simulink model "testFrame_ADCRawToIab"  (R2020b)
settings: Solver=VariableStepAuto  StartTime=0.0  StopTime=10.0  RelTol=1e-3
settings Model: Creator=unix  LastModifiedBy=unix

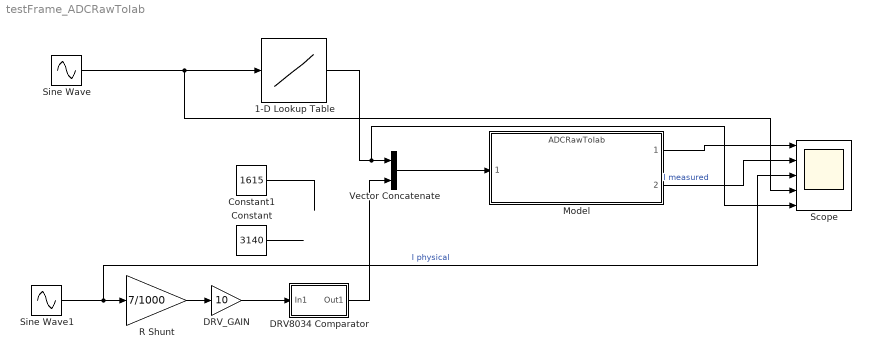
== system testFrame_ADCRawToIab ==
  1-D Lookup Table : Lookup_n-D  NumberOfTableDimensions=1  LookupTableObject=''  BreakpointsForDimension1=[0 3.3]  BreakpointsForDimension1FirstPoint=10  BreakpointsForDimension2FirstPoint=10  BreakpointsForDimension1Spacing=12  BreakpointsForDimension2Spacing=12  Table=[0 4096]  ExtrapMethod=Clip  DiagnosticForOutOfRangeInput=Error  InternalRulePriority=Speed  OutDataTypeStr=Inherit: Inherit via back propagation  RndMeth=Simplest  InputSameDT=on
  Constant : Constant  Value=3140  OutDataTypeStr=uint16
  Constant1 : Constant  Value=1615  OutDataTypeStr=uint16
  DRV8034 Comparator : Subsystem
  DRV_GAIN : Gain  Gain=10
  Model : ModelReference  ModelNameDialog=ADCRawToIab.slx  ModelReferenceVersion=3.1
  R Shunt : Gain  Gain=7/1000
  Scope : Scope  NumInputPorts=5
  Sine Wave : Sin  Amplitude=1.65  Bias=1.65  Frequency=50  SampleTime=0
  Sine Wave1 : Sin  Amplitude=22  Frequency=50  SampleTime=0
  Vector Concatenate : Concatenate
  wires:
  Sine Wave/1 -> Scope/4, 1-D Lookup Table/1
  Vector Concatenate/1 -> Model/1
  Model/1 -> Scope/1
  Model/2 -> Scope/2  "I measured"
  1-D Lookup Table/1 -> Vector Concatenate/1, Scope/5
  Sine Wave1/1 -> Scope/3, R Shunt/1  "I physical"
  R Shunt/1 -> DRV_GAIN/1
  DRV_GAIN/1 -> DRV8034 Comparator/1(In1)
  Constant/1 -> ?
  DRV8034 Comparator/1(Out1) -> Vector Concatenate/2
  Constant1/1 -> ?

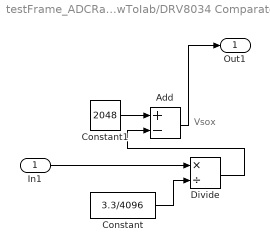
== system testFrame_ADCRawToIab/DRV8034 Comparator ==
  note: Vsox
  In1 : Inport
  Add : Sum  Inputs=+-  OutDataTypeStr=uint16
  Constant : Constant  Value=3.3/4096
  Constant1 : Constant  Value=2048  OutDataTypeStr=uint16
  Divide : Product  Inputs=*/  OutDataTypeStr=int16
  Out1 : Outport
  wires:
  Constant/1 -> Divide/2
  Divide/1 -> Add/2
  Constant1/1 -> Add/1
  In1/1 -> Divide/1
  Add/1 -> Out1/1
